simulink model "tests"  (Simulink 6.6)
settings: Solver=ode45  StartTime=0.0  StopTime=10.0  RelTol=1e-3
InitFcn:
  | slunit_init_fcn
libraries: slunit_lib x7, simulink x2
settings Model: Creator=bwmairs  LastModifiedBy=bwmairs
settings DebuggingCC: SolverPrmCheckMsg=none

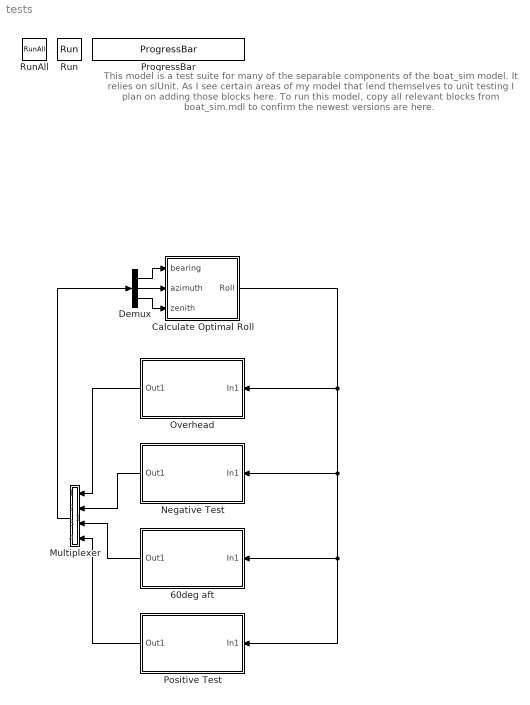
== system tests ==
  note: This model is a test suite for many of the separable components of the boat_sim model.
      | It relies on slUnit. As I see certain areas of my model that lend themselves to unit testing
      | I plan on adding those blocks here.
      |
      | To run this model, copy all relevant blocks from boat_sim.mdl to confirm the newest
      | versions are here.
  60deg aft : Subsystem  Orientation=left
      settings: CopyFcn=set_param(gcb, 'LinkStatus', 'none');
      mask Type: SLUNIT_TEST
  Calculate Optimal Roll : Subsystem
  Demux : Demux  Outputs=3
  Multiplexer : Subsystem  Orientation=left  AncestorBlock=slunit_lib/Multiplexer/Multiplexer  mask(SLUNIT_MULTIPLEXER){signals=3, inputs=4, select=4}
      mask prompts: signals "Number of Signals"
      mask help: Switches between all connected tests.
      mask init:
      | slunit_create_multiplexer(gcb, inputs);
      mask Display: disp('')
  Negative Test : Subsystem  Orientation=left
      settings: CopyFcn=set_param(gcb, 'LinkStatus', 'none');
      mask Type: SLUNIT_TEST
  Overhead : Subsystem  Orientation=left
      settings: CopyFcn=set_param(gcb, 'LinkStatus', 'none');
      mask Type: SLUNIT_TEST
  Positive Test : Subsystem  Orientation=left
      settings: CopyFcn=set_param(gcb, 'LinkStatus', 'none');
      mask Type: SLUNIT_TEST
  ProgressBar : slunit_lib/Basic/ProgressBar  SystemSampleTime=-1
  Run : slunit_lib/Basic/Run  SystemSampleTime=-1
  RunAll : slunit_lib/Basic/RunAll  SystemSampleTime=-1
  wires:
  Multiplexer/1(out) -> Demux/1
  Overhead/1(Out1) -> Multiplexer/1(in1)
  Calculate Optimal Roll/1(Roll) -> Overhead/1(In1), Negative Test/1(In1), 60deg aft/1(In1), Positive Test/1(In1)
  Demux/2 -> Calculate Optimal Roll/2(azimuth)
  Demux/1 -> Calculate Optimal Roll/1(bearing)
  Demux/3 -> Calculate Optimal Roll/3(zenith)
  Negative Test/1(Out1) -> Multiplexer/2(in2)
  60deg aft/1(Out1) -> Multiplexer/3(in3)
  Positive Test/1(Out1) -> Multiplexer/4(in4)

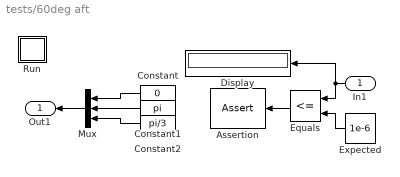
== system tests/60deg aft ==
  In1 : Inport  Orientation=left
  Assertion : slunit_lib/Assertions/Assert  Orientation=left  SystemSampleTime=-1  active=0
  Constant : Constant  Orientation=left  Value=0
  Constant1 : Constant  Orientation=left  Value=pi
  Constant2 : Constant  Orientation=left  Value=pi/3
  Display : Display
  Equals : RelationalOperator  Orientation=left  Operator=<=  LogicOutDataTypeMode=Boolean
  Expected : Constant  Orientation=left  Value=1e-6  OutDataTypeMode=double
  Mux : Mux  Orientation=left  Inputs=3
  Run : Subsystem
      settings: OpenFcn=slunit_start(bdroot, 2, gcs)
      mask Type: SLUNIT_START
      mask Display: color('white'); disp('>')
  Out1 : Outport  Orientation=left
  wires:
  Constant1/1 -> Mux/2
  Constant2/1 -> Mux/3
  Constant/1 -> Mux/1
  Mux/1 -> Out1/1
  Equals/1 -> Assertion/1
  Expected/1 -> Equals/2
  In1/1 -> Display/1, Equals/1

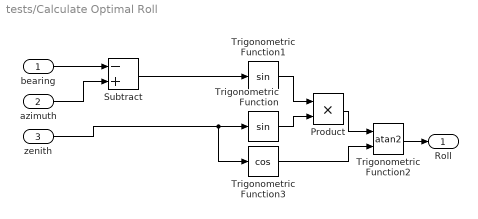
== system tests/Calculate Optimal Roll ==
  bearing : Inport
  azimuth : Inport  Port=2
  zenith : Inport  Port=3
  Product : Product  RndMeth=Zero
  Subtract : Sum  Inputs=-+  OutScaling=2^-10
  Trigonometric Function : Trigonometry
  Trigonometric Function1 : Trigonometry
  Trigonometric Function2 : Trigonometry  Operator=atan2
  Trigonometric Function3 : Trigonometry  Operator=cos
  Roll : Outport
  wires:
  Trigonometric Function/1 -> Product/2
  Trigonometric Function1/1 -> Product/1
  Product/1 -> Trigonometric Function2/1
  Trigonometric Function3/1 -> Trigonometric Function2/2
  Subtract/1 -> Trigonometric Function1/1
  bearing/1 -> Subtract/1
  azimuth/1 -> Subtract/2
  zenith/1 -> Trigonometric Function/1, Trigonometric Function3/1
  Trigonometric Function2/1 -> Roll/1

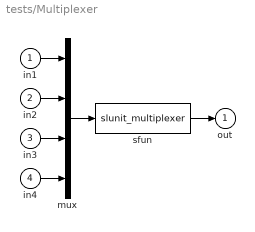
== system tests/Multiplexer ==
  in1 : Inport
  in2 : Inport  Port=2
  in3 : Inport  Port=3
  in4 : Inport  Port=4
  mux : Mux
  sfun : S-Function  FunctionName=slunit_multiplexer  Parameters=select,signals
  out : Outport
  wires:
  sfun/1 -> out/1
  in1/1 -> mux/1
  mux/1 -> sfun/1
  in2/1 -> mux/2
  in3/1 -> mux/3
  in4/1 -> mux/4

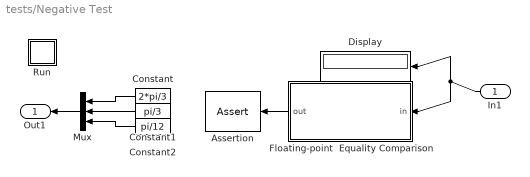
== system tests/Negative Test ==
  In1 : Inport  Orientation=left
  Assertion : slunit_lib/Assertions/Assert  Orientation=left  SystemSampleTime=-1  active=0
  Constant : Constant  Orientation=left  Value=2*pi/3
  Constant1 : Constant  Orientation=left  Value=pi/3
  Constant2 : Constant  Orientation=left  Value=pi/12
  Display : Display
  Floating-point  Equality Comparison : Subsystem  Orientation=left  mask{tolerance=1e-4, compareValue=-0.228}
      mask prompts: compareValue "Value to compare to"
      mask Display: text(0.5,0.5, '==')
  Mux : Mux  Orientation=left  Inputs=3
  Run : Subsystem
      settings: OpenFcn=slunit_start(bdroot, 2, gcs)
      mask Type: SLUNIT_START
      mask Display: color('white'); disp('>')
  Out1 : Outport  Orientation=left
  wires:
  Constant1/1 -> Mux/2
  Constant2/1 -> Mux/3
  Constant/1 -> Mux/1
  Mux/1 -> Out1/1
  Floating-point  Equality Comparison/1(out) -> Assertion/1
  In1/1 -> Display/1, Floating-point  Equality Comparison/1(in)

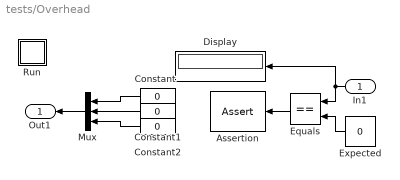
== system tests/Overhead ==
  In1 : Inport  Orientation=left
  Assertion : slunit_lib/Assertions/Assert  Orientation=left  SystemSampleTime=-1  active=0
  Constant : Constant  Orientation=left  Value=0
  Constant1 : Constant  Orientation=left  Value=0
  Constant2 : Constant  Orientation=left  Value=0
  Display : Display
  Equals : RelationalOperator  Orientation=left  Operator===  LogicOutDataTypeMode=Boolean
  Expected : Constant  Orientation=left  Value=0
  Mux : Mux  Orientation=left  Inputs=3
  Run : Subsystem
      settings: OpenFcn=slunit_start(bdroot, 2, gcs)
      mask Type: SLUNIT_START
      mask Display: color('white'); disp('>')
  Out1 : Outport  Orientation=left
  wires:
  In1/1 -> Equals/1, Display/1
  Expected/1 -> Equals/2
  Equals/1 -> Assertion/1
  Mux/1 -> Out1/1
  Constant/1 -> Mux/1
  Constant2/1 -> Mux/3
  Constant1/1 -> Mux/2

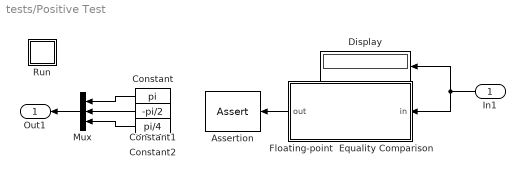
== system tests/Positive Test ==
  In1 : Inport  Orientation=left
  Assertion : slunit_lib/Assertions/Assert  Orientation=left  SystemSampleTime=-1  active=0
  Constant : Constant  Orientation=left  Value=pi
  Constant1 : Constant  Orientation=left  Value=-pi/2
  Constant2 : Constant  Orientation=left  Value=pi/4
  Display : Display
  Floating-point  Equality Comparison : Subsystem  Orientation=left  mask{tolerance=1e-4, compareValue=pi/4}
      mask prompts: compareValue "Value to compare to"
      mask Display: text(0.5,0.5, '==')
  Mux : Mux  Orientation=left  Inputs=3
  Run : Subsystem
      settings: OpenFcn=slunit_start(bdroot, 2, gcs)
      mask Type: SLUNIT_START
      mask Display: color('white'); disp('>')
  Out1 : Outport  Orientation=left
  wires:
  In1/1 -> Floating-point  Equality Comparison/1(in), Display/1
  Floating-point  Equality Comparison/1(out) -> Assertion/1
  Mux/1 -> Out1/1
  Constant/1 -> Mux/1
  Constant2/1 -> Mux/3
  Constant1/1 -> Mux/2

== system tests/60deg aft/Run ==

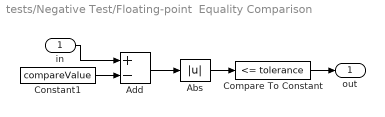
== system tests/Negative Test/Floating-point  Equality Comparison ==
  in : Inport
  Abs : Abs
  Add : Sum  Inputs=+-  OutScaling=2^-10
  Compare To Constant : simulink/Logic and Bit Operations/Compare To Constant  SystemSampleTime=-1  relop=<=  const=tolerance  LogicOutDataTypeMode=boolean  ZeroCross=off
  Constant1 : Constant  Value=compareValue
  out : Outport
  wires:
  Constant1/1 -> Add/2
  Add/1 -> Abs/1
  Abs/1 -> Compare To Constant/1
  in/1 -> Add/1
  Compare To Constant/1 -> out/1

== system tests/Negative Test/Run ==

== system tests/Overhead/Run ==

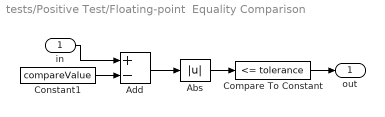
== system tests/Positive Test/Floating-point  Equality Comparison ==
  in : Inport
  Abs : Abs
  Add : Sum  Inputs=+-  OutScaling=2^-10
  Compare To Constant : simulink/Logic and Bit Operations/Compare To Constant  SystemSampleTime=-1  relop=<=  const=tolerance  LogicOutDataTypeMode=boolean  ZeroCross=off
  Constant1 : Constant  Value=compareValue
  out : Outport
  wires:
  Compare To Constant/1 -> out/1
  in/1 -> Add/1
  Abs/1 -> Compare To Constant/1
  Add/1 -> Abs/1
  Constant1/1 -> Add/2

== system tests/Positive Test/Run ==
